simulink model "mini_project_simul"  (R2021a)
settings: Solver=VariableStepAuto  StartTime=0.0  StopTime=10.0  RelTol=1e-3
settings Model: Creator=zmartinez  LastModifiedBy=zmartinez

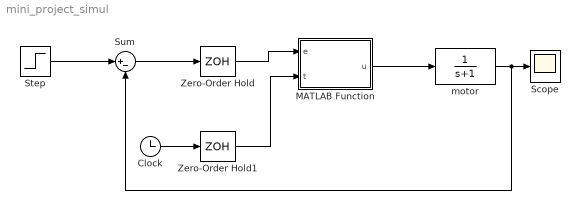
== system mini_project_simul ==
  "Clock " : Clock
  "MATLAB Function " : MATLAB Function  TreatAsAtomicUnit=on
  "Scope " : Scope
  "Step " : Step  SampleTime=0
  Sum : Sum  Inputs=|+-
  "Zero-Order Hold " : ZeroOrderHold  SampleTime=-1
  "Zero-Order Hold1 " : ZeroOrderHold  SampleTime=-1
  motor : TransferFcn  Denominator=[1 1]
  wires:
  "Step "/1 -> Sum/1
  Sum/1 -> "Zero-Order Hold "/1
  "Zero-Order Hold "/1 -> "MATLAB Function "/1(e)
  "Clock "/1 -> "Zero-Order Hold1 "/1
  "Zero-Order Hold1 "/1 -> "MATLAB Function "/2(t)
  "MATLAB Function "/1(u) -> motor/1
  motor/1 -> Sum/2, "Scope "/1

== matlab function mini_project_simul/MATLAB Function  ==
  data: e input; u output; t input
function u = fcn(e,t)
%% Define Variables
% Control Gains
Kp=.5;
Ki=0.04;
umax = 10;
% Memory variables
persistent I_past;
persistent t_past;
if isempty(I_past), I_past=0; end;
if isempty(t_past), t_past=0; end;
%% Calculate Controller output
% sample time
Ts = t - t_past;
% Integrator
I = I_past+e*Ts;
% PI control calculation

u = Kp*e+Ki*I;
% anti-windup
if abs(u)>umax,
u = sign(u)*umax;
e = sign(e)*min(umax/Kp, abs(e));
I = (u-Kp*e)/Ki;
end;
I_past=I;
t_past=t;
